simulink model "sf_fromworkspace"  (Simulink 7.6)
settings: Solver=ode45  StartTime=0.0  StopTime=100  MaxStep=.1  RelTol=1e-3
PreLoadFcn:
  | eval('load r12mlworkspace')
undefined symbols (not defined in the file or in its folder): delay, gain
CloseFcn:
  | evalin('base','clear delay gain;')
settings Model: Creator=The MathWorks Inc.  CovMetricSettings=dcmtr  ExtModeAutoUpdateStatusClock=off
settings DataIOCC: SaveTime=off  SignalLoggingName=sigsOut
settings OptimizationCC: BooleanDataType=off  InlineInvariantSignals=on  InitFltsAndDblsToZero=on  EfficientMapNaN2IntZero=off
settings DebuggingCC: SaveWithParameterizedLinksMsg=none  SignalResolutionControl=TryResolveAllWithWarning  SolverPrmCheckMsg=none  MultiTaskDSMMsg=warning  MultiTaskCondExecSysMsg=none  StrictBusMsg=None
settings HardwareCC: TargetUnknown=on
settings SFSimCC: SimParseCustomCode=off
settings RTWCC: IncludeERTFirstTime=on
settings GRTTargetCC: TargetFcnLib=ansi_tfl_tmw.mat

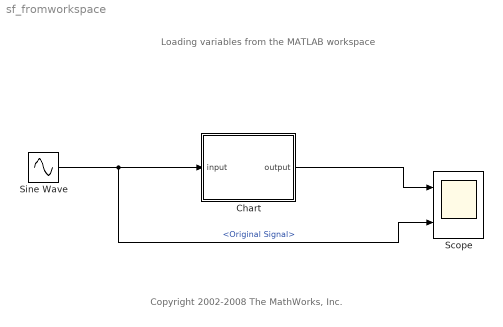
== system sf_fromworkspace ==
  note: Loading variables from the MATLAB workspace
  note: Copyright 2002-2008 The MathWorks, Inc.
  Chart : Stateflow chart  TreatAsAtomicUnit=on
  Scope : Scope  NumInputPorts=2
      settings: TimeRange=100  YMin=-5~-1  YMax=5~1
  Sine Wave : Sin  SampleTime=0
  wires:
  Sine Wave/1 -> Chart/1(input), Scope/2  "<Original Signal>"
  Chart/1(output) -> Scope/1

== stateflow chart Chart ==
  state A
    output=0;
  state B
    du: output=gain*input;
  note: The following variables are initialized
      | from the MATLAB workspace:
      |
      | gain    =  5
      | delay   =  20 (in seconds)
  A -> B : [t>delay]
  (default) -> A
  data: gain local double; input input double; output output double; delay local double
